simulink model "SystemHIL"  (R2025a)
settings: Solver=VariableStepAuto  StartTime=0.0  StopTime=10.0  RelTol=1e-3
undefined symbols (not defined in the file): Down, Pull, w_max
libraries: speedgoatlib_IO691 x4, canmsglib x3, ESys x1, autolibshared x1
settings Model: DataDictionary=System.sldd  Creator=tecnicomcbti  LastModifiedBy=tecnicomcbti

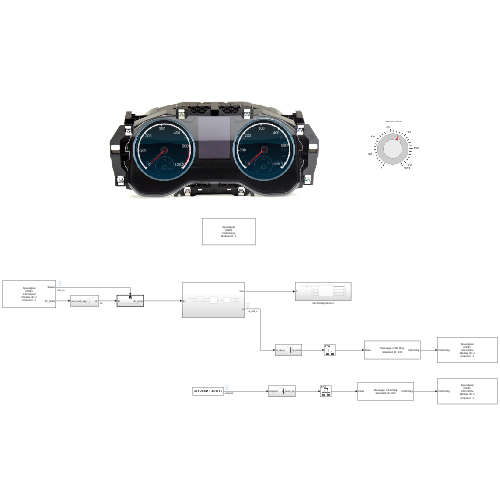
[thumbnail: Simulink's stored preview of the top-level diagram]
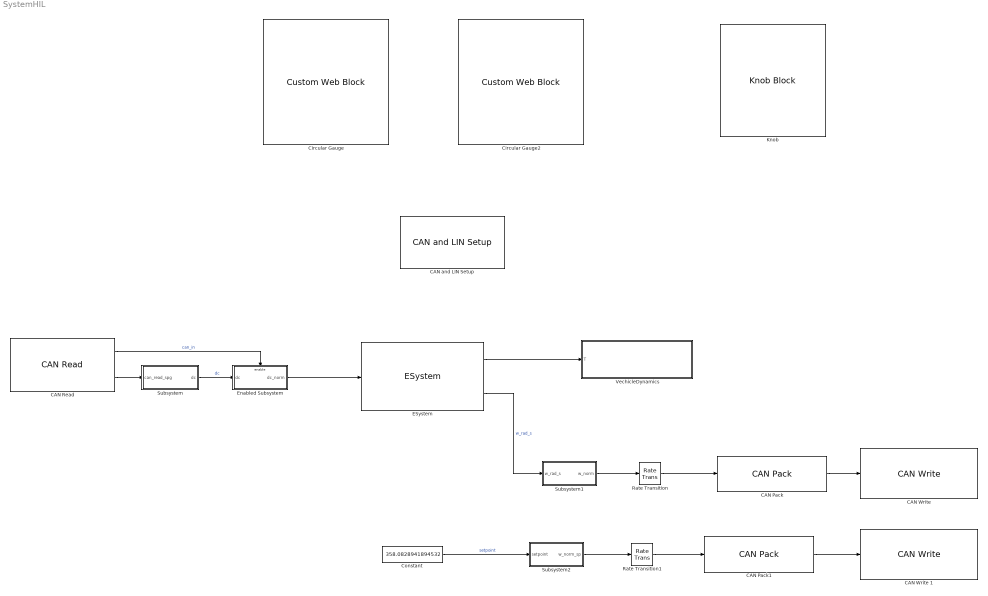
== system SystemHIL ==
  CAN Pack : canmsglib/CAN Pack  MsgList=(none)  MsgName=CAN Msg  MsgIDType=Standard (11-bit identifier)  MsgIdentifier=100  CANIDInput=off  MsgLength=8  Remote=off  ApplyMinMax=off  BusOutput=off  SignalInfo={}
      settings: DataFormat=raw data
  CAN Pack1 : canmsglib/CAN Pack  MsgList=(none)  MsgName=CAN Msg  MsgIDType=Standard (11-bit identifier)  MsgIdentifier=300  CANIDInput=off  MsgLength=8  Remote=off  ApplyMinMax=off  BusOutput=off  SignalInfo={}
      settings: DataFormat=raw data
  "CAN Read " : speedgoatlib_IO691/CAN Read   moduleType=IO691  id=1  channel=1  messageType=CAN (HS)  useBusOut=off  HasMulRead=Specify by IDs  MsgIDlist=250  isEFF=off  LabelInHex=on  enableInput=off  initValues=[691 1 0.01 0 1 0 0 2 0 1 250]  ts=10e-3
      settings: SourceProductName=IO691
  "CAN Write " : speedgoatlib_IO691/CAN Write   moduleType=IO691  id=1  channel=1  messageType=CAN (HS)  useBusIn=off  numOfMsg=1  enableInput=off  enableStatusPort=off  ts=10e-3  initValues=[691 1 0.01 0 1 0 1 0 0]
      settings: SourceProductName=IO691
  CAN Write 1 : speedgoatlib_IO691/CAN Write   moduleType=IO691  id=1  channel=1  messageType=CAN (HS)  useBusIn=off  numOfMsg=1  enableInput=off  enableStatusPort=off  ts=10e-3  initValues=[691 1 0.01 0 1 0 1 0 0]
      settings: SourceProductName=IO691
  "CAN and LIN Setup " : speedgoatlib_IO691/CAN and LIN Setup   moduleInitValues="[691    1    1   -1   -1]"  id=1  moduleType=IO691  pciSlot=-1  canChn1=CAN (HS)  canChn2=CAN (HS)  canChn3=Disabled  canChn4=Disabled  linChn1=Disabled  linChn2=Disabled  canInitStructArray=[]  canTermStructArray=[]  gpioChnx=Disabled  canChn1InitValues="[2   2   8   1  16   3  19   2   2   5   2   0]"  arbBdrChn1=500 kBaud  clockDividerChn1=Enable  arbManBdrChn1=[8,1,16,3]  fdBdrChn1=5.0 MBaud  fdManBdrChn1=[2,2,5,2]  termResistor1=off  canChn2InitValues="[2   2   8   1  16   3  19   2   2   5   2   0]"  arbBdrChn2=500 kBaud  clockDividerChn2=Enable  arbManBdrChn2=[8,1,16,3]  fdBdrChn2=5.0 MBaud  fdManBdrChn2=[2,2,5,2]  termResistor2=off  canChn3InitValues="[1   0   2   8  31   8  19   2   2   5   2   0]"  arbBdrChn3=1.0 MBaud  clockDividerChn3=Enable  arbManBdrChn3=[2,8,31,8]  fdBdrChn3=5.0 MBaud  fdManBdrChn3=[2,2,5,2]  termResistor3=off  canChn4InitValues="[1   0   2   8  31   8  19   2   2   5   2   0]"  arbBdrChn4=1.0 MBaud  clockDividerChn4=Enable  arbManBdrChn4=[2,8,31,8]  fdBdrChn4=5.0 MBaud  fdManBdrChn4=[2,2,5,2]  termResistor4=off  linChn1InitValues="[0  9600]"  linBtrChn1=9600  linChn2InitValues="[0  9600]"  linBtrChn2=9600  doInitTermStruct="[0  5  0  0  0]"  parDoChannels=[1 2]  parDoVoltage=5  parDoInitValues=0  parDoReset=1  parNumOfDoS=0  parDiChannels=[3 4]  parDiVoltage=5  parDiPull=Pull-Down
      settings: SourceProductName=IO691
  Circular Gauge : CustomWebBlock  LabelPosition=Hide  ShowInitialText=on  Configuration="{\"components\":[{\"name\":\"CircularScaleComponent\",\"settings\":{\"bounds\":{\"max\":628.32,\"min\":0,\"tickInterval\":100},\"direction\":\"cw\",\"flipLimits\":0,\"innerRadius\":0.84,\"internalTickHeightScaleFactor\":1,\"labelColor\":[255,255,255],\"labelFont\":{\"font\":\"Arial\",\"fontSize\":12},\"labelRadius\":0.73,\"labelTransparency\":1,\"minorTickHeightScaleFactor\":0.2,\"needleImage\":{\"size\":[200,50],\"src\":\"data:image\\/svg+xml;base64,PD94bWwgdmVyc2lvbj0iMS4wIiBlbmNvZGluZz0idXRmLTgiPz4KPCEtLSBHZW5lcmF0b3I6IEFkb2JlIElsbHVzdHJhdG9yIDI0LjEuMiwgU1ZHIEV4cG9ydCBQbHVnLUluIC4gU1ZHIFZlcnNpb246IDYuMDAgQnVpbGQgMCkgIC0tPgo8c3ZnIHZlcnNpb249IjEuMSIgaWQ9IkxheWVyXzEiIHhtbG5zPSJodHRwOi8vd3d3LnczLm9yZy8yMDAwL3N2ZyIgeG1sbnM6eGxpbms9Imh0dHA6Ly93d3cudzMub3JnLzE5OTkveGxpbmsiIHg9IjBweCIgeT0iMHB4IgoJIHZpZXdCb3g9IjAgMCAyMDAgNTAiIHN0eWxlPSJlbmFibGUtYmFja2dyb3VuZDpuZXcgMCAwIDIwMCA1MDsiIHhtbDpzcGFjZT0icHJlc2VydmUiPgo8c3R5bGUgdHlwZT0idGV4dC9jc3MiPgoJLnN0MHtmaWxsOiNFQzIxMjc7fQo8L3N0eWxlPgo8cGF0aCBjbGFzcz0ic3QwIiBkPSJNMTYyLjgsMTMuN0MxNjksNC40LDE4MS43LDEuOSwxOTEsOC4xczExLjgsMTguOSw1LjYsMjguMnMtMTguOSwxMS44LTI4LjIsNS42bDAsMAoJQzE1OS4xLDM1LjYsMTU2LjYsMjMsMTYyLjgsMTMuN0wxNjIuOCwxMy43eiBNMTY1LjgsMTUuOGMtNS4xLDcuNi0zLjEsMTcuOSw0LjYsMjNjNy42LDUuMSwxNy45LDMuMSwyMy00LjYKCWM1LjEtNy42LDMuMS0xNy45LTQuNi0yM2wwLDBDMTgxLjIsNi4yLDE3MC45LDguMiwxNjUuOCwxNS44eiIvPgo8cGF0aCBjbGFzcz0ic3QwIiBkPSJNMC40LDI1Ljl2LTMuM2wxNTktMi41Yy0wLjcsMi42LTAuNyw1LjIsMCw3LjhMMC40LDI1Ljl6Ii8+CjxjaXJjbGUgY2xhc3M9InN0MCIgY3g9IjE3OS42IiBjeT0iMjQiIHI9IjAuNyIvPgo8L3N2Zz4K\"},\"needleOffset\":[0.14813151041666667,0],\"needleOrientation\":-45,\"needleRotation\":180,\"needleSize\":{\"height\":0.099,\"width\":0.379},\"outerRadius\":0.9,\"position\":[0.057291666666666664,0.057291666666666664,0.8999837239583334,0.8999837239583334],\"referencePoint\":\"auto\",\"scaleAngle\":270,\"scaleAngleOffset\":135,\"scaleColors\":[{\"Color\":[162,20,47],\"Max\":628.32,\"Min\":500}],\"scaleColorsSize\":0.2,\"scaleDirection\":\"CW\",\"scalePosition\":[0,0,1,1],\"showLabels\":1,\"showMinorTicks\":1,\"showSpanLine\":1,\"showTicks\":1,\"tickColor\":[255,255,255],\"tickTransparency\":1,\"valueBarColor\":[0,114,189],\"valueBarPosition\":[0,0,1,1],\"valueBarSize\":0.2,\"valueBarTransparency\":1}},{\"name\":\"BackgroundImageComponent\",\"settings\":{\"image\":{\"size\":[500,500],\"src\":\"data:image\\/svg+xml;base64,PD94bWwgdmVyc2lvbj0iMS4wIiBlbmNvZGluZz0iVVRGLTgiIHN0YW5kYWxvbmU9Im5vIj8+CjxzdmcKICAgeG1sbnM6ZGM9Imh0dHA6Ly9wdXJsLm9yZy9kYy9lbGVtZW50cy8xLjEvIgogICB4bWxuczpjYz0iaHR0cDovL2NyZWF0aXZlY29tbW9ucy5vcmcvbnMjIgogICB4bWxuczpyZGY9Imh0dHA6Ly93d3cudzMub3JnLzE5OTkvMDIvMjItcmRmLXN5bnRheC1ucyMiCiAgIHhtbG5zOnN2Zz0iaHR0cDovL3d3dy53My5vcmcvMjAwMC9zdmciCiAgIHhtbG5zPSJodHRwOi8vd3d3LnczLm9yZy8yMDAwL3N2ZyIKICAgeG1sbnM6 ...(+9964 chars)\"},\"position\":[0,0,1,1],\"scaleMode\":\"0\"}},{\"name\":\"ForegroundImageComponent\",\"settings\":{\"image\":{\"size\":[0,0],\"src\":\"default\",\"srcOrientation\":[]},\"isForeground\":1,\"position\":[0,0,1,1],\"scaleMode\":\"0\"}}],\"derived\":{\"blockParameters\":{\"ForegroundColor\":[1,1,1],\"Limits\":{\"Max\":628.32,\"Min\":0,\"Ticks\":100},\"ScaleColors\":[{\"Color\":[162,20,47],\"Max\":628.32,\"Min\":500}],\"ScaleDirection\":\"Clockwise\",\"ScaleMax\":628.32,\"ScaleMin\":0,\"TickInterval\":100,\"fixedAspectRatio\":\"on\"}},\"settings\":{\"BindingType\":\"signal\",\"aspectRatio\":1.032258064516129,\"backgroundColor\":[0,0,0,\"1\"],\"backgroundOffset\":1,\"backgroundOpacity\":1,\"direction\":\"cw\",\"fixedAspectRatio\":\"on\",\"flipLimits\":0,\"orientation\":\"horizontal\",\"showBackgroundColor\":false,\"value\":0,\"version\":\"R2023a\"},\"type\":\"CircularGauge\"}"
  Circular Gauge2 : CustomWebBlock  LabelPosition=Hide  ShowInitialText=on  Configuration="{\"components\":[{\"name\":\"CircularScaleComponent\",\"settings\":{\"bounds\":{\"max\":628.32,\"min\":0,\"tickInterval\":100},\"direction\":\"cw\",\"flipLimits\":0,\"innerRadius\":0.84,\"internalTickHeightScaleFactor\":1,\"labelColor\":[255,255,255],\"labelFont\":{\"font\":\"Arial\",\"fontSize\":12},\"labelRadius\":0.72,\"labelTransparency\":1,\"minorTickHeightScaleFactor\":0.2,\"needleImage\":{\"size\":[200,50],\"src\":\"data:image\\/svg+xml;base64,PD94bWwgdmVyc2lvbj0iMS4wIiBlbmNvZGluZz0idXRmLTgiPz4KPCEtLSBHZW5lcmF0b3I6IEFkb2JlIElsbHVzdHJhdG9yIDI0LjEuMiwgU1ZHIEV4cG9ydCBQbHVnLUluIC4gU1ZHIFZlcnNpb246IDYuMDAgQnVpbGQgMCkgIC0tPgo8c3ZnIHZlcnNpb249IjEuMSIgaWQ9IkxheWVyXzEiIHhtbG5zPSJodHRwOi8vd3d3LnczLm9yZy8yMDAwL3N2ZyIgeG1sbnM6eGxpbms9Imh0dHA6Ly93d3cudzMub3JnLzE5OTkveGxpbmsiIHg9IjBweCIgeT0iMHB4IgoJIHZpZXdCb3g9IjAgMCAyMDAgNTAiIHN0eWxlPSJlbmFibGUtYmFja2dyb3VuZDpuZXcgMCAwIDIwMCA1MDsiIHhtbDpzcGFjZT0icHJlc2VydmUiPgo8c3R5bGUgdHlwZT0idGV4dC9jc3MiPgoJLnN0MHtmaWxsOiNFQzIxMjc7fQo8L3N0eWxlPgo8cGF0aCBjbGFzcz0ic3QwIiBkPSJNMTYyLjgsMTMuN0MxNjksNC40LDE4MS43LDEuOSwxOTEsOC4xczExLjgsMTguOSw1LjYsMjguMnMtMTguOSwxMS44LTI4LjIsNS42bDAsMAoJQzE1OS4xLDM1LjYsMTU2LjYsMjMsMTYyLjgsMTMuN0wxNjIuOCwxMy43eiBNMTY1LjgsMTUuOGMtNS4xLDcuNi0zLjEsMTcuOSw0LjYsMjNjNy42LDUuMSwxNy45LDMuMSwyMy00LjYKCWM1LjEtNy42LDMuMS0xNy45LTQuNi0yM2wwLDBDMTgxLjIsNi4yLDE3MC45LDguMiwxNjUuOCwxNS44eiIvPgo8cGF0aCBjbGFzcz0ic3QwIiBkPSJNMC40LDI1Ljl2LTMuM2wxNTktMi41Yy0wLjcsMi42LTAuNyw1LjIsMCw3LjhMMC40LDI1Ljl6Ii8+CjxjaXJjbGUgY2xhc3M9InN0MCIgY3g9IjE3OS42IiBjeT0iMjQiIHI9IjAuNyIvPgo8L3N2Zz4K\"},\"needleOffset\":[0.18,0],\"needleOrientation\":-45,\"needleRotation\":180,\"needleSize\":{\"height\":0.11741692305346914,\"width\":0.46108337545091255},\"outerRadius\":0.9,\"position\":[0.05,0.05,0.9,0.9],\"referencePoint\":\"auto\",\"scaleAngle\":270,\"scaleAngleOffset\":135,\"scaleColors\":[],\"scaleColorsSize\":0.2,\"scaleDirection\":\"CW\",\"scalePosition\":[0,0,1,1],\"showLabels\":1,\"showMinorTicks\":1,\"showSpanLine\":true,\"showTicks\":1,\"tickColor\":[255,255,255],\"tickTransparency\":1,\"valueBarColor\":[0,114,189],\"valueBarPosition\":[0,0,1,1],\"valueBarSize\":0.2,\"valueBarTransparency\":1}},{\"name\":\"BackgroundImageComponent\",\"settings\":{\"image\":{\"size\":[500,500],\"src\":\"data:image\\/svg+xml;base64,PD94bWwgdmVyc2lvbj0iMS4wIiBlbmNvZGluZz0iVVRGLTgiIHN0YW5kYWxvbmU9Im5vIj8+CjxzdmcKICAgeG1sbnM6ZGM9Imh0dHA6Ly9wdXJsLm9yZy9kYy9lbGVtZW50cy8xLjEvIgogICB4bWxuczpjYz0iaHR0cDovL2NyZWF0aXZlY29tbW9ucy5vcmcvbnMjIgogICB4bWxuczpyZGY9Imh0dHA6Ly93d3cudzMub3JnLzE5OTkvMDIvMjItcmRmLXN5bnRheC1ucyMiCiAgIHhtbG5zOnN2Zz0iaHR0cDovL3d3dy53My5vcmcvMjAwMC9zdmciCiAgIHhtbG5zPSJodHRwOi8vd3d3LnczLm9yZy8yMDAwL3N2ZyIKICAgeG1sbnM6 ...(+9964 chars)\"},\"position\":[0,0,1,1],\"scaleMode\":\"0\"}},{\"name\":\"ForegroundImageComponent\",\"settings\":{\"image\":{\"size\":[0,0],\"src\":\"default\",\"srcOrientation\":[]},\"isForeground\":1,\"position\":[0,0,1,1],\"scaleMode\":\"0\"}}],\"derived\":{\"blockParameters\":{\"ForegroundColor\":[1,1,1],\"Limits\":{\"Max\":628.32,\"Min\":0,\"Ticks\":100},\"ScaleColors\":[],\"ScaleDirection\":\"Clockwise\",\"ScaleMax\":628.32,\"ScaleMin\":0,\"TickInterval\":100,\"fixedAspectRatio\":\"on\"}},\"settings\":{\"BindingType\":\"signal\",\"aspectRatio\":1.032258064516129,\"backgroundColor\":[0,0,0,\"1\"],\"backgroundOffset\":1,\"backgroundOpacity\":1,\"direction\":\"cw\",\"fixedAspectRatio\":\"on\",\"flipLimits\":0,\"orientation\":\"horizontal\",\"showBackgroundColor\":false,\"value\":0,\"version\":\"R2023a\"},\"type\":\"CircularGauge\"}"
  Constant : Constant  Value=358.0828941894532
  ESystem : ESys/ESystem  SystemSampleTime=-1  VariantActivationTime=update diagram  EmptyChoice=off  PassThrough=off  PassThroughVariantControl=(default)  EmptyChoiceVariantControl=(default)  AllowFlexibleInterface=on  Latency=0  AutoFrameSizeCalculation=off
  Enabled Subsystem : Subsystem  TreatAsAtomicUnit=on
  Knob : KnobBlock  ScaleMax=628.32  TickInterval=100
  Rate Transition : RateTransition
  Rate Transition1 : RateTransition
  Subsystem : Subsystem
  Subsystem1 : Subsystem
  Subsystem2 : Subsystem
  VechicleDynamics : Subsystem
  wires:
  "CAN Read "/1 -> Enabled Subsystem/Enable  "can_in"
  Subsystem/1(dc) -> Enabled Subsystem/1(dc)  "dc"
  "CAN Read "/2 -> Subsystem/1(can_read_spg)
  Enabled Subsystem/1(dc_norm) -> ESystem/1
  Rate Transition1/1 -> CAN Pack1/1
  Rate Transition/1 -> CAN Pack/1
  Subsystem2/1(w_norm_sp) -> Rate Transition1/1
  CAN Pack1/1 -> CAN Write 1/1
  Constant/1 -> Subsystem2/1(setpoint)  "setpoint"
  ESystem/2 -> Subsystem1/1(w_rad_s)  "w_rad_s"
  CAN Pack/1 -> "CAN Write "/1
  Subsystem1/1(w_norm) -> Rate Transition/1
  ESystem/1 -> VechicleDynamics/1(T)

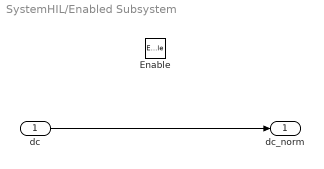
== system SystemHIL/Enabled Subsystem ==
  dc : Inport
  Enable : EnablePort
  dc_norm : Outport
  wires:
  dc/1 -> dc_norm/1

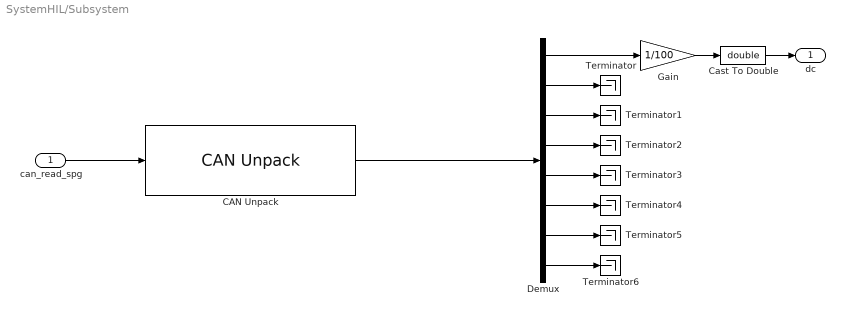
== system SystemHIL/Subsystem ==
  can_read_spg : Inport
  CAN Unpack : canmsglib/CAN Unpack  MsgList=(none)  MsgName=CAN Msg  MsgIDType=Standard (11-bit identifier)  MsgIdentifier=250  MsgLength=8  SignalInfo={}  IDPort=off  TimestampPort=off  ErrorPort=off  RemotePort=off  LengthPort=off  StatusPort=off  ApplyMinMax=off
      settings: DataFormat=raw data
  Cast To Double : DataTypeConversion  OutDataTypeStr=double  SaturateOnIntegerOverflow=off  RndMeth=Floor
  Demux : Demux  Outputs=8
  Gain : Gain  Gain=1/100
  Terminator{,1..6} (7 alike) : Terminator
  dc : Outport
  wires:
  Gain/1 -> Cast To Double/1
  CAN Unpack/1 -> Demux/1
  can_read_spg/1 -> CAN Unpack/1
  Cast To Double/1 -> dc/1
  Demux/8 -> Terminator6/1
  Demux/7 -> Terminator5/1
  Demux/6 -> Terminator4/1
  Demux/5 -> Terminator3/1
  Demux/4 -> Terminator2/1
  Demux/3 -> Terminator1/1
  Demux/2 -> Terminator/1
  Demux/1 -> Gain/1

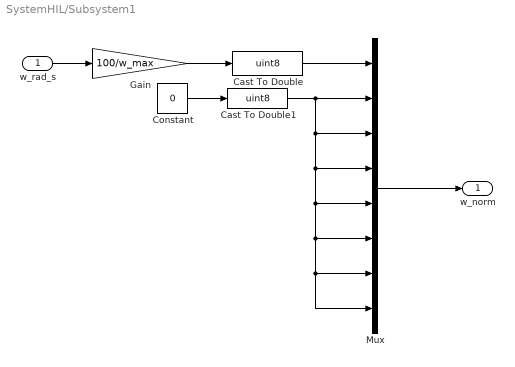
== system SystemHIL/Subsystem1 ==
  w_rad_s : Inport
  Cast To Double : DataTypeConversion  OutDataTypeStr=uint8  SaturateOnIntegerOverflow=off  RndMeth=Floor
  Cast To Double1 : DataTypeConversion  OutDataTypeStr=uint8  SaturateOnIntegerOverflow=off  RndMeth=Floor
  Constant : Constant  Value=0
  Gain : Gain  Gain=100/w_max
  Mux : Mux  Inputs=8
  w_norm : Outport
  wires:
  Gain/1 -> Cast To Double/1
  Mux/1 -> w_norm/1
  Cast To Double1/1 -> Mux/2, Mux/3, Mux/4, Mux/5, Mux/6, Mux/7, Mux/8
  Constant/1 -> Cast To Double1/1
  Cast To Double/1 -> Mux/1
  w_rad_s/1 -> Gain/1

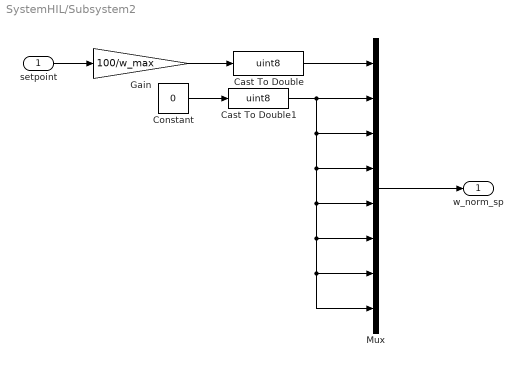
== system SystemHIL/Subsystem2 ==
  setpoint : Inport
  Cast To Double : DataTypeConversion  OutDataTypeStr=uint8  SaturateOnIntegerOverflow=off  RndMeth=Floor
  Cast To Double1 : DataTypeConversion  OutDataTypeStr=uint8  SaturateOnIntegerOverflow=off  RndMeth=Floor
  Constant : Constant  Value=0
  Gain : Gain  Gain=100/w_max
  Mux : Mux  Inputs=8
  w_norm_sp : Outport
  wires:
  setpoint/1 -> Gain/1
  Cast To Double/1 -> Mux/1
  Constant/1 -> Cast To Double1/1
  Cast To Double1/1 -> Mux/8, Mux/7, Mux/6, Mux/5, Mux/4, Mux/3, Mux/2
  Mux/1 -> w_norm_sp/1
  Gain/1 -> Cast To Double/1

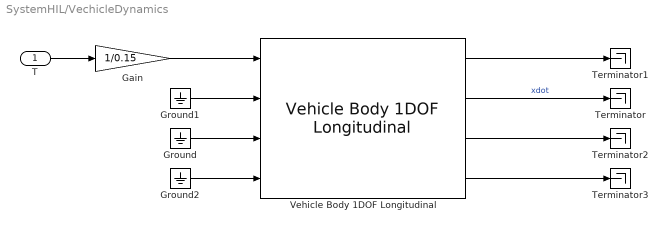
== system SystemHIL/VechicleDynamics ==
  T : Inport
  Gain : Gain  Gain=1/0.15
  Ground : Ground
  Ground1 : Ground
  Ground2 : Ground
  Terminator{,1..3} (4 alike) : Terminator
  Vehicle Body 1DOF Longitudinal : autolibshared/Vehicle Body 1DOF Longitudinal  VariantControl=SL  extFMode=off  extMMode=off  extTamb=off  wind3D=off  aMode=2  NF=2  NR=2  m=50  a=.4  b=.8  h=.6  Cd=.6  Cl=0  Cpm=0  Af=0.15  x_o=0  xdot_o=0  Pabs=101325  T=273  g=9.81
      settings: LibrarySourceBlock=vehdynlibeom/Vehicle Body 1DOF Longitudinal
  wires:
  Vehicle Body 1DOF Longitudinal/4 -> Terminator3/1
  Vehicle Body 1DOF Longitudinal/3 -> Terminator2/1
  Vehicle Body 1DOF Longitudinal/1 -> Terminator1/1
  Ground2/1 -> Vehicle Body 1DOF Longitudinal/4
  Ground1/1 -> Vehicle Body 1DOF Longitudinal/2
  Ground/1 -> Vehicle Body 1DOF Longitudinal/3
  Vehicle Body 1DOF Longitudinal/2 -> Terminator/1  "xdot"
  T/1 -> Gain/1
  Gain/1 -> Vehicle Body 1DOF Longitudinal/1
